simulink model "SecRwRtStChldLckChk"  (R2018b)
settings: Solver=FixedStepDiscrete  StartTime=0.0  StopTime=10.0  FixedStep=0.01  RelTol=1e-3
undefined symbols (not defined in the file or in its folder): SeatChldLkSt
settings Model: Creator=sn2xws  LastModifiedBy=sn2xws
settings DataIOCC: SaveFormat=StructureWithTime
settings OptimizationCC: DefaultParameterBehavior=Inlined  EnhancedBackFolding=on  PassReuseOutputArgsAs=Individual arguments  ZeroExternalMemoryAtStartup=off  ZeroInternalMemoryAtStartup=off  OptimizeBlockOrder=speed  DifferentSizesBufferReuse=on  OptimizationCustomize=off
settings DebuggingCC: ParameterTunabilityLossMsg=error
settings ModelReferenceCC: ModelReferenceNumInstancesAllowed=Single
settings SFSimCC: MATLABDynamicMemAlloc=off
settings RTWCC: SystemTargetFile=autosar.tlc  GenCodeOnly=on  TemplateMakefile=ert_default_tmf  Description=AUTOSAR  GenerateReport=on  IncludeHyperlinkInReport=on  LaunchReport=on  GenerateTraceInfo=on  GenerateTraceReport=on  GenerateTraceReportSl=on  GenerateTraceReportSf=on  GenerateTraceReportEml=on
settings CodeAppCC: ForceParamTrailComments=on  IgnoreCustomStorageClasses=off  OperatorAnnotations=on  SimulinkDataObjDesc=on  SFDataObjDesc=on  InsertBlockDesc=on
settings STFCustomTargetCC: TargetLangStandard=C99 (ISO)  MultiwordLength=256  ParMdlRefBuildCompliant=on  CompOptLevelCompliant=on  IncludeMdlTerminateFcn=off  CombineOutputUpdateFcns=on  SuppressErrorStatus=on  ERTCustomFileBanners=on  SupportNonFinite=off  SupportComplex=off  SupportContinuousTime=off  SupportNonInlinedSFcns=off  RemoveResetFunc=on  MATLABClassNameForMDSCustomization=Simulink.SoftwareTarget.ERTCustomization  AutosarCompliant=on  UseToolchainInfoCompliant=on  LookupTableObjectStructAxisOrder=2,1,3,4,...  LUTObjectStructOrderEvenSpacing=Size,Table,Breakpoints  SystemTargetFile=autosar.tlc
settings ERTTargetCC: TargetLangStandard=C99 (ISO)  ConcurrentExecutionCompliant=off  IncludeMdlTerminateFcn=off  SuppressErrorStatus=on  SupportNonFinite=off  SupportComplex=off  ModelStepFunctionPrototypeControlCompliant=off  CPPClassGenCompliant=off  AutosarCompliant=on  LookupTableObjectStructAxisOrder=2,1,3,4,...  LUTObjectStructOrderEvenSpacing=Size,Table,Breakpoints  InlinedParameterPlacement=NonHierarchical  ERTCustomFileTemplate=example_file_process.tlc  ERTFilePackagingFormat=Compact

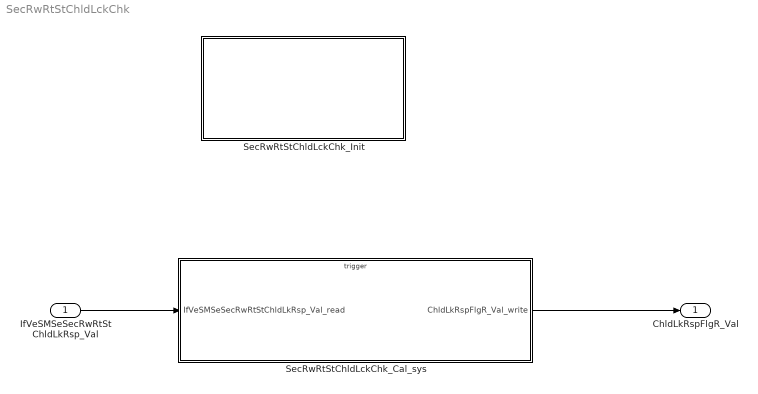
== system SecRwRtStChldLckChk ==
  IfVeSMSeSecRwRtStChldLkRsp_Val : Inport  OutDataTypeStr=Enum: SeatChldLkSt  PortDimensions=1
  SecRwRtStChldLckChk_Cal_sys : Subsystem
  SecRwRtStChldLckChk_Init : Subsystem
  ChldLkRspFlgR_Val : Outport  OutDataTypeStr=boolean  PortDimensions=1
  wires:
  IfVeSMSeSecRwRtStChldLkRsp_Val/1 -> SecRwRtStChldLckChk_Cal_sys/1(IfVeSMSeSecRwRtStChldLkRsp_Val_read)
  SecRwRtStChldLckChk_Cal_sys/1(ChldLkRspFlgR_Val_write) -> ChldLkRspFlgR_Val/1

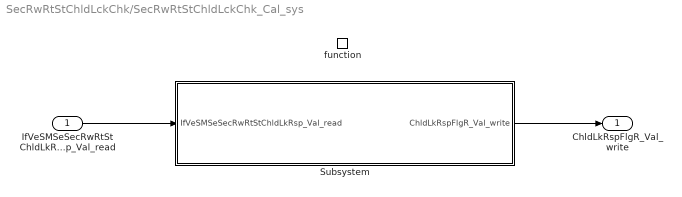
== system SecRwRtStChldLckChk/SecRwRtStChldLckChk_Cal_sys ==
  IfVeSMSeSecRwRtStChldLkRsp_Val_read : Inport
  function : TriggerPort  TriggerType=function-call  IsSimulinkFunction=on  FunctionName=SecRwRtStChldLckChk_Cal  VariantControl=(inherit)
  Subsystem : Subsystem
  ChldLkRspFlgR_Val_write : Outport
      settings: EnsureOutportIsVirtual=on
  wires:
  IfVeSMSeSecRwRtStChldLkRsp_Val_read/1 -> Subsystem/1(IfVeSMSeSecRwRtStChldLkRsp_Val_read)
  Subsystem/1(ChldLkRspFlgR_Val_write) -> ChldLkRspFlgR_Val_write/1

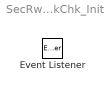
== system SecRwRtStChldLckChk/SecRwRtStChldLckChk_Init ==
  Event Listener : EventListener  EventName=reset

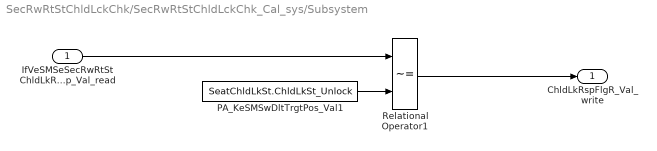
== system SecRwRtStChldLckChk/SecRwRtStChldLckChk_Cal_sys/Subsystem ==
  IfVeSMSeSecRwRtStChldLkRsp_Val_read : Inport
  PA_KeSMSwDltTrgtPos_Val1 : Constant  Value=SeatChldLkSt.ChldLkSt_Unlock
  Relational Operator1 : RelationalOperator  Operator=~=  OutDataTypeStr=boolean  RndMeth=Simplest
  ChldLkRspFlgR_Val_write : Outport
      settings: EnsureOutportIsVirtual=on
  wires:
  IfVeSMSeSecRwRtStChldLkRsp_Val_read/1 -> Relational Operator1/1
  PA_KeSMSwDltTrgtPos_Val1/1 -> Relational Operator1/2
  Relational Operator1/1 -> ChldLkRspFlgR_Val_write/1
